simulink model "ANC"  (R2021b)
settings: Solver=FixedStepDiscrete  StartTime=0.0  StopTime=10  RelTol=1e-3
libraries: dspsnks4 x1, dspadpt3 x1, dspvision x1, dspindex x1
settings Model: Creator=The MathWorks, Inc.  LastModifiedBy=Shera
settings SolverCC: AlgebraicLoopSolver=TrustRegion
settings DataIOCC: ReturnWorkspaceOutputs=off
settings DebuggingCC: SFMachineParentedDataDiag=warning  ArithmeticOperatorsInVariantConditions=warning
settings SFSimCC: CustomCodeUndefinedFunction=UseInterfaceOnly

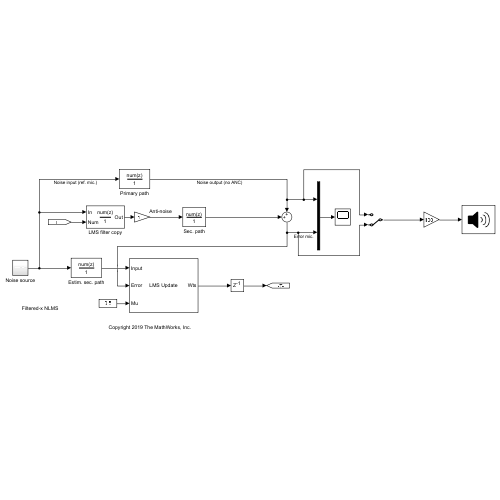
[thumbnail: Simulink's stored preview of the top-level diagram]
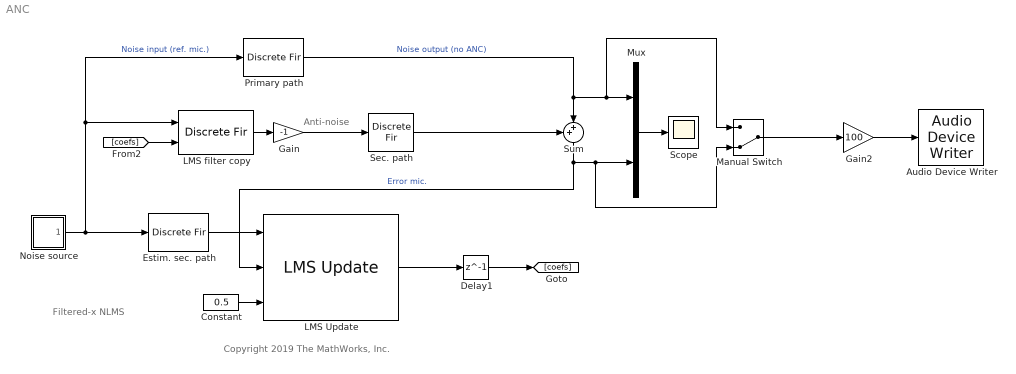
== system ANC ==
  note: Filtered-x NLMS
  note: Anti-noise
  note: Copyright 2019 The MathWorks, Inc.
  Audio Device Writer : dspsnks4/Audio Device Writer  Driver=DirectSound  Device=Default  InheritSampleRate=on  SampleRate=44100  BitDepth=16-bit integer  BufferSize=4096  NumBuffers=10  DefaultOutputChannelMapping=on  OutputChannelMapping=1:2  OutputNumUnderrunSamples=off  DriverIdx=1  DeviceWarnFlag=''
  Constant : Constant  Value=0.5
  Delay1 : Delay  DelayLength=1
  Estim. sec. path : DiscreteFir  Coefficients=[0.2 0.02 0.1 -.02 -.03 -0.01]
  Gain : Gain  Gain=-1
  Gain2 : Gain  Gain=100
  LMS Update : dspadpt3/LMS Update  Method=Normalized LMS  Length=24  StepSizeSource=Input port  StepSize=0.1  LeakageFactor=1.0  InitialConditions=0  EnableAdaptInput=off  EnableResetInput=off  SimulateUsing=Interpreted execution
      settings: SourceProductBaseCode=DS
  LMS filter copy : DiscreteFir  CoefSource=Input port
      settings: InputPortMap=u0,u1
  Manual Switch : ManualSwitch  CurrentSetting=0
  Mux : Mux  Inputs=2
  Noise source : Subsystem
  Primary path : DiscreteFir  Coefficients=conv([0.02 0.02 0.1 -.02 -.03 -0.01],[.1 -.1 .2 -.2 .3 -.3 .15 -.15])
  Scope : Scope
  Sec. path : DiscreteFir  Coefficients=[0.2 0.02 0.1 -.02 -.03 -0.01]
  Sum : Sum  Inputs=++|
  wires:
  Primary path/1 -> Manual Switch/1, Mux/1, Sum/2  "Noise output (no ANC)"
  LMS filter copy/1 -> Gain/1
  Sum/1 -> LMS Update/2, Manual Switch/2, Mux/2  "Error mic."
  Estim. sec. path/1 -> LMS Update/1
  Mux/1 -> Scope/1
  LMS Update/1 -> Delay1/1
  Noise source/1(Out1) -> Estim. sec. path/1, LMS filter copy/1, Primary path/1  "Noise input (ref. mic.)"
  Constant/1 -> LMS Update/3
  Delay1/1 -> [coefs]
  Gain/1 -> Sec. path/1
  Sec. path/1 -> Sum/1
  Manual Switch/1 -> Gain2/1
  [coefs] -> LMS filter copy/2
  Gain2/1 -> Audio Device Writer/1

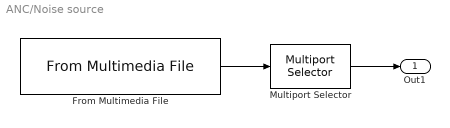
== system ANC/Noise source ==
  From Multimedia File : dspvision/From Multimedia File  inputFilename=Noise.wav  readRange=[1 Inf]  loop=on  numPlays=inf  outputStreams=Audio only  videoDataType=single  audioDataType=double  inheritSampleTime=on  userDefinedSampleTime=1/22050  noAudioOutput=off  isIntensityVideo=off  fourcc=RGB  colorVideoFormat=Separate color signals  outputEOF=off  dataOrg=Column-major  audioFrameSize=1  computeAudioFrameSize=off  outSamplingMode=Sample based
  Multiport Selector : dspindex/Multiport Selector  rowsOrCols=Columns  idxCellArray=1  idxErrMode=Clip Index
  Out1 : Outport  VectorParamsAs1DForOutWhenUnconnected=off
  wires:
  Multiport Selector/1 -> Out1/1
  From Multimedia File/1 -> Multiport Selector/1
